simulink model "Tut2_2014a"  (R2014a)
settings: Solver=ode45  SolverMode=SingleTasking  StartTime=0.0  StopTime=2  RelTol=1e-3
libraries: simulink x1
settings Model: CovMetricSettings=dwe  CovHtmlReporting=off  covSaveCumulativeToWorkspaceVar=off  CovSaveSingleToWorkspaceVar=off  CovExternalEMLEnable=on  CovSFcnEnable=on  Creator=Gu  LastModifiedBy=duong
settings DataIOCC: LimitDataPoints=off  SaveFormat=StructureWithTime
settings DebuggingCC: MergeDetectMultiDrivingBlocksExec=error  SolverPrmCheckMsg=none  FrameProcessingCompatibilityMsg=error  SFUnexpectedBacktrackingDiag=error  SFNoUnconditionalDefaultTransitionDiag=error
settings HardwareCC: ProdBitPerPointer=64  ProdLargestAtomicFloat=Float  ProdIntDivRoundTo=Zero  ProdEndianess=LittleEndian  ProdHWDeviceType=Specified
settings ModelReferenceCC: PropagateSignalLabelsOutOfModel=on
settings SFSimCC: SimUseLocalCustomCode=on
settings RTWCC: RTWUseLocalCustomCode=on
settings GRTTargetCC: TargetLangStandard=C99 (ISO)

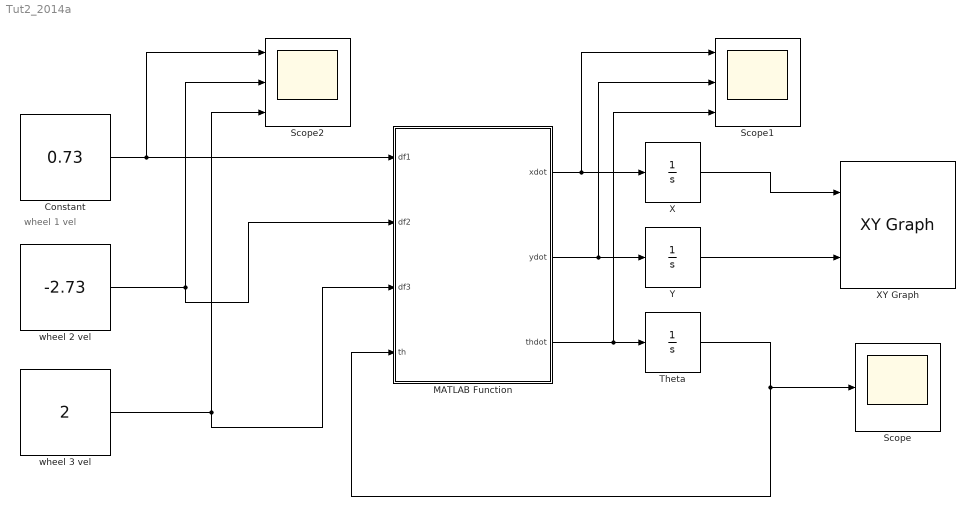
== system Tut2_2014a ==
  note: wheel 1 vel
  Constant : Constant  Value=0.73
  MATLAB Function : MATLAB Function  TreatAsAtomicUnit=on
      settings: PermitHierarchicalResolution=ParametersOnly
  Scope : Scope
      settings: TimeRange=auto  MaxDataPoints=5000  SaveToWorkspace=off  SaveName=ScopeData  YMin=-1.00000  YMax=1.00000  SampleTime=-1
  Scope1 : Scope  NumInputPorts=3
      settings: TimeRange=auto  MaxDataPoints=5000  SaveToWorkspace=off  YMin=-0.125~-5~-5  YMax=1.125~5~5  SampleTime=-1
  Scope2 : Scope  NumInputPorts=3
      settings: TimeRange=auto  MaxDataPoints=5000  SaveToWorkspace=off  SaveName=ScopeData2  YMin=-3.32125~-5~-5  YMax=2.59125~5~5  SampleTime=-1
  Theta : Integrator
  X : Integrator
  XY Graph : simulink/Sinks/XY Graph  xmin=-5  xmax=5  ymin=-5  ymax=5  st=-1
  Y : Integrator
  wheel 2 vel : Constant  Value=-2.73
  wheel 3 vel : Constant  Value=2
  wires:
  Constant/1 -> Scope2/1, MATLAB Function/1(df1)
  wheel 2 vel/1 -> MATLAB Function/2(df2), Scope2/2
  wheel 3 vel/1 -> MATLAB Function/3(df3), Scope2/3
  MATLAB Function/1(xdot) -> Scope1/1, X/1
  MATLAB Function/2(ydot) -> Scope1/2, Y/1
  MATLAB Function/3(thdot) -> Scope1/3, Theta/1
  X/1 -> XY Graph/1
  Y/1 -> XY Graph/2
  Theta/1 -> Scope/1, MATLAB Function/4(th)

== matlab function Tut2_2014a/MATLAB Function ==
  data: df1 input; xdot output; df2 input; df3 input; ydot output; thdot output; th input
function [xdot,ydot,thdot] = swedish_w(df1,df2,df3,th)
% in this function df1, df2 and df3 are the 3 wheels rotation velocity
%
l=2;
% the pure rolling constraints for 3 wheels.
pr=[sqrt(3)/2 -0.5 -l;-sqrt(3)/2 -0.5 -l;0 1 -l];

% the rotation matrix between robot frame and fixed frame is depending on
% the heading angle of the robot - th.
R=[cos(th) sin(th) 0;-sin(th) cos(th) 0;0 0 1];

% assuming wheel radius is 0.5m

r=0.5;

vr=[r*df1;r*df2;r*df3]; % wheels linear velocity

% the robot velocity in fixed frame is:
VF = R^-1*pr^-1*vr;
xdot=VF(1);
ydot=VF(2);
thdot=VF(3);
